simulink model "untitled"  (R2021b)
settings: Solver=FixedStepDiscrete  StartTime=0.0  StopTime=10  FixedStep=5e-4  RelTol=1e-3
settings Model: PauseTimes=2.4  SnapshotBufferSize=50  SnapshotInterval=50  Creator=KURAPAS  LastModifiedBy=KURAPAS

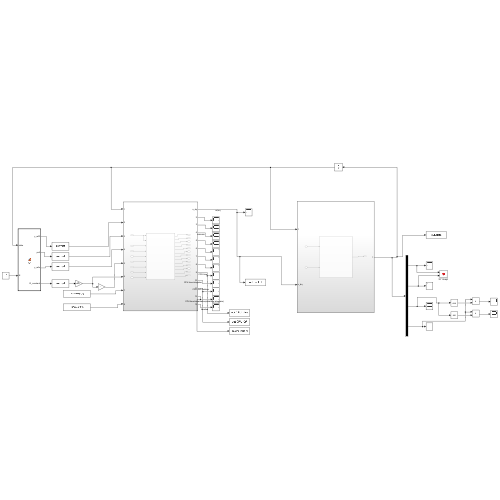
[thumbnail: Simulink's stored preview of the top-level diagram]
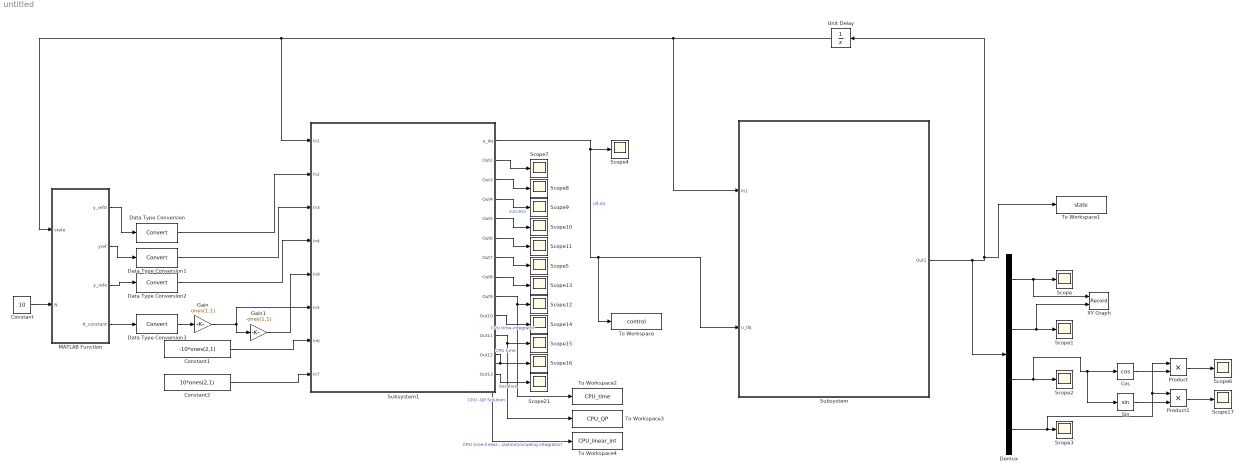
== system untitled ==
  Constant : Constant  Value=10
  Constant1 : Constant  Value=-10*ones(2,1)
  Constant2 : Constant  Value=10*ones(2,1)
  Cos : Trigonometry  Operator=cos
  Data Type Conversion{,1..3} (4 alike) : DataTypeConversion
  Demux : Demux
  Gain : Gain  Gain=ones(1,1)
  Gain1 : Gain  Gain=-ones(1,1)
  MATLAB Function : MATLAB Function  TreatAsAtomicUnit=on
  Product : Product
  Product1 : Product
  Scope{,1..17,21} (19 alike) : Scope
  Sin : Trigonometry
  Subsystem : Subsystem
  Subsystem1 : Subsystem
  To Workspace : ToWorkspace  VariableName=control  SampleTime=-1
  To Workspace1 : ToWorkspace  VariableName=state  SampleTime=-1
  To Workspace2 : ToWorkspace  VariableName=CPU_time  SampleTime=-1
  To Workspace3 : ToWorkspace  VariableName=CPU_QP  SampleTime=-1
  To Workspace4 : ToWorkspace  VariableName=CPU_linear_int  SampleTime=-1
  Unit Delay : UnitDelay  InitialCondition=[0; 0; pi/4; 60]  SampleTime=-1  HasFrameUpgradeWarning=on
  XY Graph : Record  FileSettingsInternal="{\"entries\":[{\"content\":{\"excelSettings\":{\"content\":{},\"type\":\"Streamout.ExcelSettings\"}},\"type\":\"Streamout.FileSettingStorage\",\"uuid\":\"cd73450b-8a4a-4fdc-844f-850cabbd2bd1\"}],\"packageUris\":[\"http://schema.mathworks.com/mf0/streamout_blocks/R2020a\"],\"version\":\"1.0\"}"  Layout=[1 1]  SignalsInternal="{\"entries\":[{\"content\":{\"signals\":[{\"content\":{\"blockPath\":[\"untitled/XY Graph\"],\"channel\":[],\"dimensions\":[1],\"domain\":\"untitled/XY Graph\",\"lineColor\":\"#a2142f\",\"plots\":[1],\"port\":1,\"sid\":[\"\"],\"signalID\":1611,\"signalName\":\"Demux:1\"},\"type\":\"RecordBlkView.Signal\",\"uuid\":\"b2324ed1-e827-4406-bb6e-bedc158c9b91\"},{\"content\":{\"blockPath\":[\"untitled/XY Graph\"],\"channel\":[],\"dimensions\":[1],\"domain\":\"untitled/XY Graph\",\"lineColor\":\"#139fff\",\"plots\":[1],\"port\":2,\"sid\":[\"\"],\"signalID\":1615,\"signalName\":\"Demux:2\"},\"type\":\"RecordBlkView.Signal\",\"uuid\":\"270ae053-ec4a-4d3b-9bc4-f00c4178dc1c\"}]},\"type\":\"RecordBlkView.InputSignals\",\"uuid\":\"e96fc8be-5457-45b2-85ae-f7a144d7fe35\"}],\"packageUris\":[\"http://schema.mathworks.com/mf0/streamout_blocks/R2020a\"],\"version\":\"1.0\"}"  VisualizationBindings="{\"xyplotplugin\":{\"info\":[{\"series\":[{\"bindingParametersList\":[{\"parameter\":\"X-Axis\",\"signalID\":1611,\"signalName\":\"Demux:1\"},{\"parameter\":\"Y-Axis\",\"signalID\":1615,\"signalName\":\"Demux:2\"}],\"seriesID\":8123}],\"subplotID\":1}]}}"  CompatibilityTag=XY
  wires:
  MATLAB Function/1(y_ref0) -> Data Type Conversion/1
  MATLAB Function/2(yref) -> Data Type Conversion1/1
  MATLAB Function/3(y_refe) -> Data Type Conversion2/1
  Subsystem1/13(Out13) -> Scope21/1  "iteration"
  Subsystem1/12(Out12) -> To Workspace4/1, Scope16/1  "CPU time-linearization(including integrator)"
  Subsystem1/11(Out11) -> Scope15/1, To Workspace3/1  "CPU -QP Solution"
  Subsystem1/10(Out10) -> Scope14/1  "CPU time-integrator"
  Subsystem1/9(Out9) -> Scope12/1, To Workspace2/1  "CPU time"
  Subsystem1/8(Out8) -> Scope13/1
  Subsystem1/7(Out7) -> Scope5/1
  Subsystem1/6(Out6) -> Scope11/1
  Subsystem1/5(Out5) -> Scope10/1
  Subsystem1/4(Out4) -> Scope9/1  "success"
  Subsystem1/3(Out3) -> Scope8/1
  Subsystem1/2(Out2) -> Scope7/1
  Subsystem/1(Out1) -> Demux/1, To Workspace1/1, Unit Delay/1
  Subsystem1/1(u_dq) -> To Workspace/1, Subsystem/2(u_dq), Scope4/1  "ud,uq"
  Unit Delay/1 -> Subsystem/1(In1), MATLAB Function/1(state), Subsystem1/1(In1)
  Demux/1 -> XY Graph/1, Scope/1
  Demux/2 -> XY Graph/2, Scope1/1
  Demux/3 -> Sin/1, Cos/1, Scope2/1
  Demux/4 -> Product1/1, Product/1, Scope3/1
  Constant/1 -> MATLAB Function/2(N)
  MATLAB Function/4(R_constant) -> Data Type Conversion3/1
  Data Type Conversion3/1 -> Gain/1
  Data Type Conversion2/1 -> Subsystem1/4(In4)
  Data Type Conversion1/1 -> Subsystem1/3(In3)
  Data Type Conversion/1 -> Subsystem1/2(In2)
  Gain/1 -> Gain1/1, Subsystem1/6(In5)
  Gain1/1 -> Subsystem1/5(In9)
  Constant1/1 -> Subsystem1/7(In6)
  Constant2/1 -> Subsystem1/8(In7)
  Cos/1 -> Product/2
  Sin/1 -> Product1/2
  Product/1 -> Scope6/1
  Product1/1 -> Scope17/1

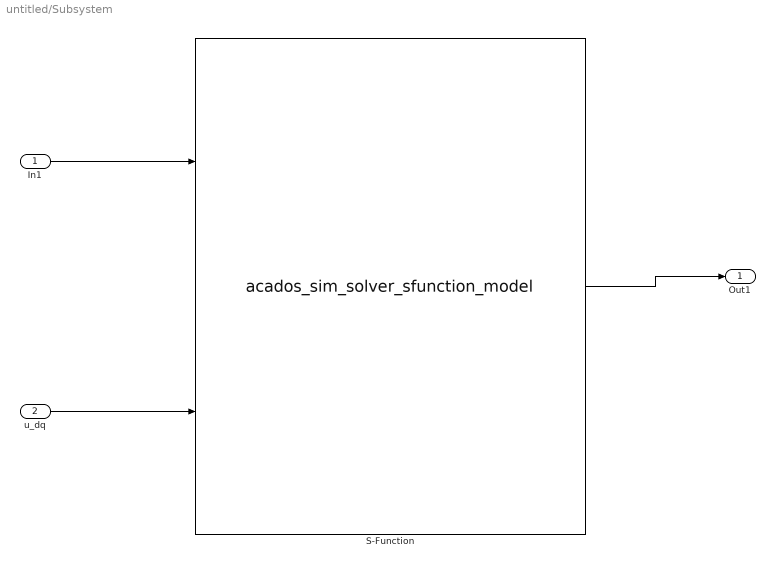
== system untitled/Subsystem ==
  In1 : Inport
  u_dq : Inport  Port=2
  S-Function : S-Function  FunctionName=acados_sim_solver_sfunction_model  SFunctionDeploymentMode=off  EnableBusSupport=off
  Out1 : Outport
  wires:
  S-Function/1 -> Out1/1
  u_dq/1 -> S-Function/2
  In1/1 -> S-Function/1

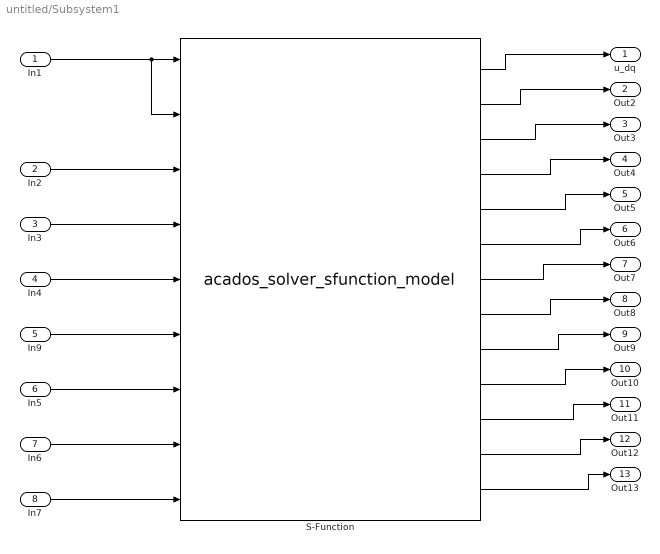
== system untitled/Subsystem1 ==
  In1 : Inport
  In2 : Inport  Port=2
  In3 : Inport  Port=3
  In4 : Inport  Port=4
  In9 : Inport  Port=5
  In5 : Inport  Port=6
  In6 : Inport  Port=7
  In7 : Inport  Port=8
  S-Function : S-Function  FunctionName=acados_solver_sfunction_model  SFunctionDeploymentMode=off  EnableBusSupport=off
  u_dq : Outport
  Out2 : Outport  Port=2
  Out3 : Outport  Port=3
  Out4 : Outport  Port=4
  Out5 : Outport  Port=5
  Out6 : Outport  Port=6
  Out7 : Outport  Port=7
  Out8 : Outport  Port=8
  Out9 : Outport  Port=9
  Out10 : Outport  Port=10
  Out11 : Outport  Port=11
  Out12 : Outport  Port=12
  Out13 : Outport  Port=13
  wires:
  In1/1 -> S-Function/2, S-Function/1
  S-Function/1 -> u_dq/1
  S-Function/2 -> Out2/1
  S-Function/3 -> Out3/1
  S-Function/4 -> Out4/1
  S-Function/5 -> Out5/1
  S-Function/6 -> Out6/1
  S-Function/7 -> Out7/1
  S-Function/8 -> Out8/1
  S-Function/9 -> Out9/1
  S-Function/10 -> Out10/1
  S-Function/11 -> Out11/1
  S-Function/12 -> Out12/1
  S-Function/13 -> Out13/1
  In5/1 -> S-Function/7
  In9/1 -> S-Function/6
  In4/1 -> S-Function/5
  In3/1 -> S-Function/4
  In2/1 -> S-Function/3
  In6/1 -> S-Function/8
  In7/1 -> S-Function/9

== matlab function untitled/MATLAB Function ==
  data: state input; y_ref0 output; N input; yref output; y_refe output; R_constant output
function [y_ref0, yref, y_refe, R_constant] = fcn(state, N)

y_ref0 = zeros(6,1);
yref = zeros(6*(2-1),1);
y_refe = zeros(4,1);
R_constant = 1e5;

x = state(1);
y = state(2);

% for i = 1:N-1
    if x <= 100 || y <= 100
        y_ref0 = [10; 10; 0; 60; 0; 0];
        yref( 1 : 6 ) = [100; 100; 0; 60; 0; 0];
        y_refe = [10; 10; 0; 60];
        R_constant = 1e5;

    elseif x < 300  ||  y < 200 
        y_ref0 = [200; 300; 0; 60; 0.5*exp(-(x-200)^2/200); 0];
        yref( 1 : 6 ) = [200; 300; 0; 60; 0.5*exp(-(x-200)^2/200); 0];
        y_refe = [200; 300; 0; 60];
        if( state(4) - 55 > 10*1e-3)
            R_constant = state(4) - 10*5e-4;
        else
            R_constant = 55;
        end
    else 
        y_ref0 = [400; 600; 0; 60; 0; 0];
        yref( 1 : 6 ) = [400; 600; 0; 60; 0; 0];
        y_refe = [400; 400; 0; 60];  
        if( state(4) - 60 > 10*1e-3)
            R_constant = state(4) + 10*5e-4;
        else
            R_constant = 60;
        end
        
%     elseif ( x >= 400 ) || ( y >= 300)
%         y_ref0 = [10, 10, 0, 60, 0, 0];
%         yref( 6*(i-1) +1 : 6*i ) = [400, 300, 0, 60, 0, 0];
%         y_refe = [10, 10, 0, 60, 0, 0];  
%         R_constant = ones(N,1) * 50;
    end
% end

end
